simulink model "whirlybird_sim"  (Simulink 8.3)
settings: Solver=ode45  StartTime=0.0  StopTime=5  RelTol=1e-3
undefined symbols (not defined in the file or in its folder): controller_whirlybird_lab2, P
settings Model: Creator=Administrator  LastModifiedBy=jhl48
settings OptimizationCC: ExpressionDepthLimit=2147483647
settings DebuggingCC: FcnCallInpInsideContextMsg=UseLocalSettings

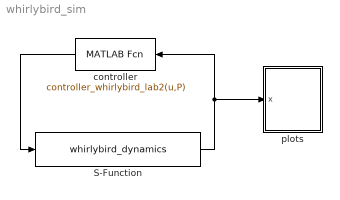
== system whirlybird_sim ==
  S-Function : S-Function  FunctionName=whirlybird_dynamics  Parameters=P  EnableBusSupport=off
  controller : MATLABFcn  MATLABFcn=controller_whirlybird_lab2(u,P)  OutputDimensions=2  SampleTime=P.Ts
  plots : Subsystem
      mask Display: image(imread('tv.jpg'))
  wires:
  S-Function/1 -> controller/1, plots/1(x)
  controller/1 -> S-Function/1

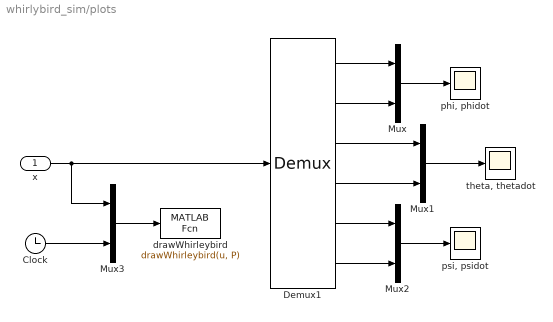
== system whirlybird_sim/plots ==
  x : Inport
  Clock : Clock
  Demux1 : Demux  Outputs=6
  Mux{,1..3} (4 alike) : Mux  Inputs=2
  drawWhirleybird : MATLABFcn  MATLABFcn=drawWhirleybird(u, P)  OutputDimensions=0  SampleTime=0.1
  "phi, phidot" : Scope
      settings: TimeRange=40  YMin=-10  YMax=15  SaveName=ScopeData4
  "psi, psidot" : Scope
      settings: TimeRange=40  YMin=-2  YMax=1  SaveName=ScopeData3
  "theta, thetadot" : Scope
      settings: TimeRange=40  YMin=-2  YMax=1  SaveName=ScopeData2
  wires:
  Demux1/1 -> Mux/1
  Demux1/2 -> Mux/2
  Demux1/3 -> Mux1/1
  Demux1/4 -> Mux1/2
  Demux1/5 -> Mux2/1
  Demux1/6 -> Mux2/2
  Mux2/1 -> "psi, psidot"/1
  Mux1/1 -> "theta, thetadot"/1
  Mux/1 -> "phi, phidot"/1
  x/1 -> Mux3/1, Demux1/1
  Clock/1 -> Mux3/2
  Mux3/1 -> drawWhirleybird/1
